simulink model "VVI"  (R2024a)
settings: Solver=FixedStepAuto  StartTime=0.0  StopTime=10.0  FixedStep=1e-3  RelTol=1e-3  EnableMultiTasking=on
undefined symbols (not defined in the file): D0, D1, D10, D11, D12, D13, D2, D3, D4, D5, D6, D7, D8, D9, PTA0, PTA1, PTA2, PTB23, PTB9, PTC16, PTC17, PTC2, PTC3, PTC4, PTD0, PTD1, PTD2, PTD3
libraries: frdmk64flib x14
settings Model: ExtModeTrigDuration=5  Creator=peter  LastModifiedBy=peter
settings OptimizationCC: EnhancedBackFolding=on  PassReuseOutputArgsAs=Individual arguments  ZeroExternalMemoryAtStartup=off  ZeroInternalMemoryAtStartup=off  MaxStackSize=64  OptimizeBlockOrder=speed  DifferentSizesBufferReuse=on  OptimizationCustomize=off  EfficientTunableParamExpr=on
settings DebuggingCC: ParameterTunabilityLossMsg=error
settings HardwareCC: ProdBitPerPointer=32  ProdBitPerSizeT=32  ProdBitPerPtrDiffT=32  ProdLargestAtomicInteger=Long  ProdLargestAtomicFloat=Double  ProdWordSize=32  ProdHWDeviceType=ARM Compatible->ARM Cortex
settings SFSimCC: MATLABDynamicMemAlloc=off
settings RTWCC: Description=Embedded Coder  SystemTargetFile=ert.tlc  HardwareBoard=NXP FRDM-K64F  TLCOptions="-aInlineSetEventsForThisBaseRateFcn=TLC_FALSE -aSuppressMultiTaskScheduler=TLC_FALSE  -aRateBasedStepFcn=0"  TemplateMakefile=ert_default_tmf  Toolchain=GNU Tools for ARM Embedded Processors
settings CodeAppCC: ForceParamTrailComments=on  IgnoreCustomStorageClasses=off  OperatorAnnotations=on  SimulinkDataObjDesc=on  SFDataObjDesc=on  InsertBlockDesc=on
settings ERTTargetCC: ExtModeTransport=4  ExtModeMexFile=sendToCommService

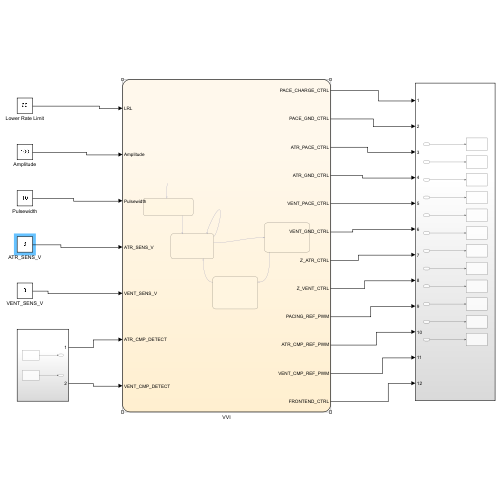
[thumbnail: Simulink's stored preview of the top-level diagram]
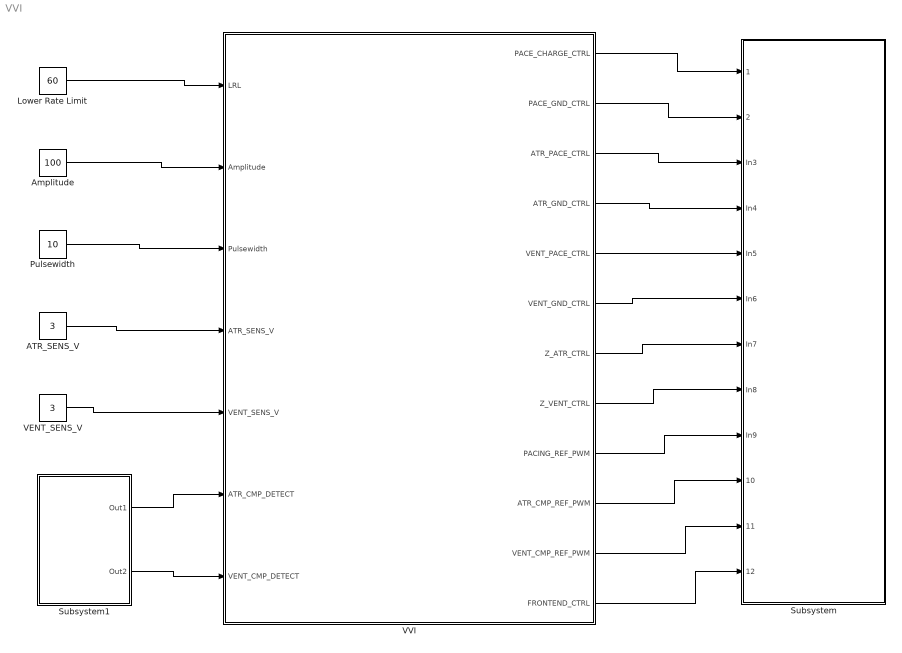
== system VVI ==
  ATR_SENS_V : Constant  Value=3
  Amplitude : Constant  Value=100
  Lower Rate Limit : Constant  Value=60
  Pulsewidth : Constant  Value=10
  Subsystem : Subsystem
  Subsystem1 : Subsystem
  VENT_SENS_V : Constant  Value=3
  VVI : Stateflow chart  TreatAsAtomicUnit=on
  wires:
  Lower Rate Limit/1 -> VVI/1(LRL)
  Amplitude/1 -> VVI/2(Amplitude)
  Pulsewidth/1 -> VVI/3(Pulsewidth)
  VVI/1(PACE_CHARGE_CTRL) -> Subsystem/1(1)
  VVI/2(PACE_GND_CTRL) -> Subsystem/2(2)
  VVI/3(ATR_PACE_CTRL) -> Subsystem/3(In3)
  VVI/4(ATR_GND_CTRL) -> Subsystem/4(In4)
  VVI/5(VENT_PACE_CTRL) -> Subsystem/5(In5)
  VVI/6(VENT_GND_CTRL) -> Subsystem/6(In6)
  VVI/7(Z_ATR_CTRL) -> Subsystem/7(In7)
  VVI/8(Z_VENT_CTRL) -> Subsystem/8(In8)
  VVI/9(PACING_REF_PWM) -> Subsystem/9(In9)
  Subsystem1/1(Out1) -> VVI/6(ATR_CMP_DETECT)
  Subsystem1/2(Out2) -> VVI/7(VENT_CMP_DETECT)
  VVI/10(ATR_CMP_REF_PWM) -> Subsystem/10(10)
  VVI/11(VENT_CMP_REF_PWM) -> Subsystem/11(11)
  VENT_SENS_V/1 -> VVI/5(VENT_SENS_V)
  ATR_SENS_V/1 -> VVI/4(ATR_SENS_V)
  VVI/12(FRONTEND_CTRL) -> Subsystem/12(12)

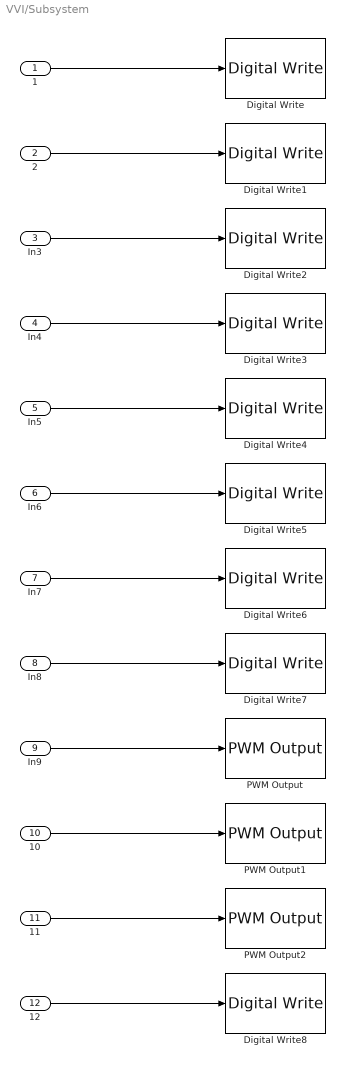
== system VVI/Subsystem ==
  1 : Inport
  2 : Inport  Port=2
  In3 : Inport  Port=3
  In4 : Inport  Port=4
  In5 : Inport  Port=5
  In6 : Inport  Port=6
  In7 : Inport  Port=7
  In8 : Inport  Port=8
  In9 : Inport  Port=9
  10 : Inport  Port=10
  11 : Inport  Port=11
  12 : Inport  Port=12
  Digital Write : frdmk64flib/Digital Write  Whichpin=PTB9 (D2)
  Digital Write1 : frdmk64flib/Digital Write  Whichpin=PTD0 (D10)
  Digital Write2 : frdmk64flib/Digital Write  Whichpin=PTA0 (D8)
  Digital Write3 : frdmk64flib/Digital Write  Whichpin=PTD2 (D11)
  Digital Write4 : frdmk64flib/Digital Write  Whichpin=PTC4 (D9)
  Digital Write5 : frdmk64flib/Digital Write  Whichpin=PTD3 (D12)
  Digital Write6 : frdmk64flib/Digital Write  Whichpin=PTB23 (D4)
  Digital Write7 : frdmk64flib/Digital Write  Whichpin=PTC3 (D7)
  Digital Write8 : frdmk64flib/Digital Write  Whichpin=PTD1 (D13)
  PWM Output : frdmk64flib/PWM Output  Whichpin=PTA2 (D5)  InitialFrequency=2000  InitialDutyCycle=100
  PWM Output1 : frdmk64flib/PWM Output  Whichpin=PTC2 (D6)  InitialFrequency=2000  InitialDutyCycle=0
  PWM Output2 : frdmk64flib/PWM Output  Whichpin=PTA1 (D3)  InitialFrequency=2000  InitialDutyCycle=0
  wires:
  1/1 -> Digital Write/1
  2/1 -> Digital Write1/1
  In3/1 -> Digital Write2/1
  In4/1 -> Digital Write3/1
  In5/1 -> Digital Write4/1
  In6/1 -> Digital Write5/1
  In7/1 -> Digital Write6/1
  In8/1 -> Digital Write7/1
  In9/1 -> PWM Output/1
  10/1 -> PWM Output1/1
  11/1 -> PWM Output2/1
  12/1 -> Digital Write8/1

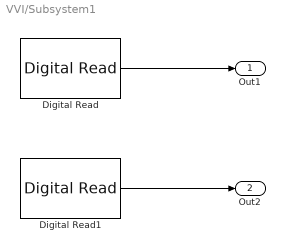
== system VVI/Subsystem1 ==
  Digital Read : frdmk64flib/Digital Read  Whichpin=PTC16 (D0)  SampleTime=-1
  Digital Read1 : frdmk64flib/Digital Read  Whichpin=PTC17 (D1)  SampleTime=-1
  Out1 : Outport
  Out2 : Outport  Port=2
  wires:
  Digital Read/1 -> Out1/1
  Digital Read1/1 -> Out2/1

== stateflow chart VVI/VVI ==
  state Initialization
    entry:
    FRONTEND_CTRL = 1;
    ATR_CMP_REF_PWM = 100*ATR_SENS_V/5
    VENT_CMP_REF_PWM = 100*VENT_SENS_V/5
  state Pacing
    entry:
    PACE_CHARGE_CTRL=0;
    PACE_GND_CTRL=1;
    ATR_PACE_CTRL=0;
    ATR_GND_CTRL=0;
    Z_ATR_CTRL=0;
    Z_VENT_CTRL=0;
    VENT_GND_CTRL=0;
    VENT_PACE_CTRL=1;
  state Charging
    entry:
    ATR_PACE_CTRL=0;
    VENT_PACE_CTRL=0;
    PACING_REF_PWM=Amplitude;
    PACE_CHARGE_CTRL=1;
  state Discharging
    entry:
    PACE_GND_CTRL=1;
    VENT_PACE_CTRL=0;
    Z_ATR_CTRL=0;
    Z_VENT_CTRL=0;
    ATR_PACE_CTRL=0;
    ATR_GND_CTRL=0;
    VENT_GND_CTRL=1;
  (default) -> Initialization
  Charging -> Charging [order 1] : after(Pulsewidth,msec)[VENT_CMP_DETECT == 1]
  Initialization -> Charging
  Charging -> Pacing [order 2] : [after((60/LRL)-(Pulsewidth/1000),sec)]
  Pacing -> Discharging : [after(Pulsewidth,msec)]
  Discharging -> Charging
  data: LRL input; Amplitude input; Pulsewidth input; ATR_SENS_V input; VENT_SENS_V input; PACE_CHARGE_CTRL output; PACE_GND_CTRL output; ATR_PACE_CTRL output; ATR_GND_CTRL output; VENT_PACE_CTRL output; VENT_GND_CTRL output; Z_ATR_CTRL output; Z_VENT_CTRL output; PACING_REF_PWM output; ATR_CMP_DETECT input; VENT_CMP_DETECT input; ATR_CMP_REF_PWM output; VENT_CMP_REF_PWM output; FRONTEND_CTRL output
